simulink model "Adaptive_Control_KpKd"  (R2021b)
settings: Solver=VariableStepAuto  StartTime=0.0  StopTime=10  RelTol=1e-3
undefined symbols (not defined in the file or in its folder): coef_init, Kd, Kp, Kpi, Lambda, q_dq_init
(part 1 of 4)
settings Model: Creator=Yafei Ou  LastModifiedBy=ouyaf

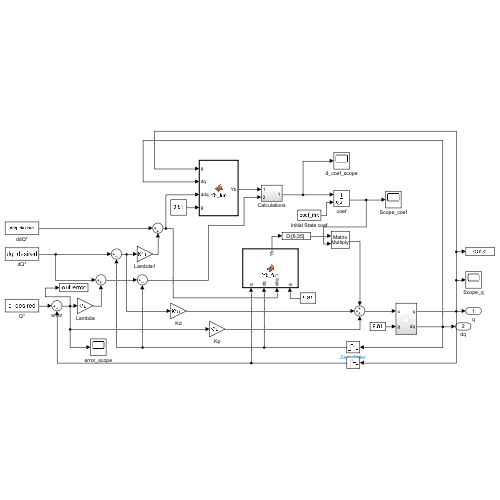
[thumbnail: Simulink's stored preview of the top-level diagram]
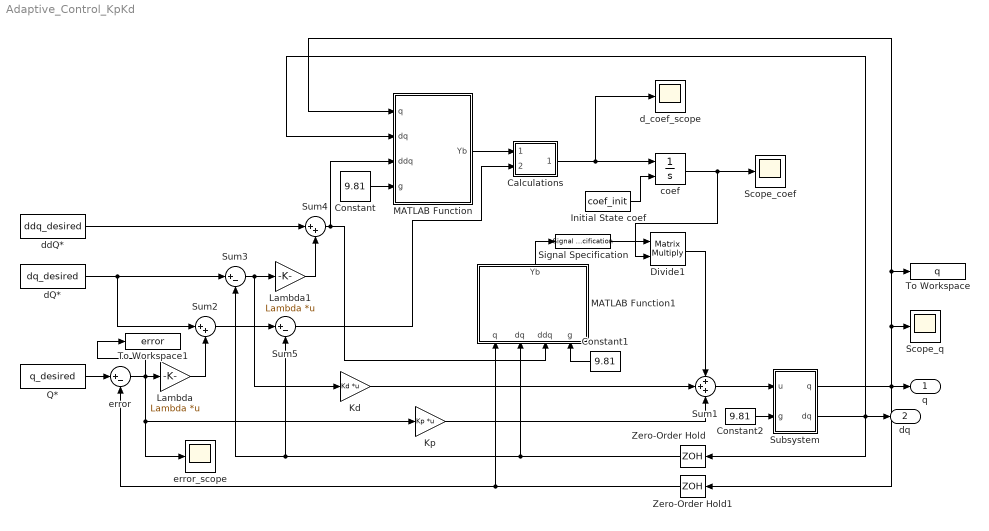
== system Adaptive_Control_KpKd ==
  Calculations : Subsystem
  Constant : Constant  Value=9.81
  Constant1 : Constant  Value=9.81
  Constant2 : Constant  Value=9.81
  Divide1 : Product  Multiplication=Matrix(*)
  Initial State coef : Constant  Value=coef_init
  Kd : Gain  Gain=Kd  Multiplication=Matrix(K*u)
  Kp : Gain  Gain=Kp  Multiplication=Matrix(K*u)
  Lambda : Gain  Gain=Lambda  Multiplication=Matrix(K*u)
  Lambda1 : Gain  Gain=Lambda  Multiplication=Matrix(K*u)
  MATLAB Function : MATLAB Function  TreatAsAtomicUnit=on
  MATLAB Function1 : MATLAB Function  TreatAsAtomicUnit=on
  Q* : FromWorkspace  VariableName=q_desired
  Scope_coef : Scope
  Scope_q : Scope
  Signal Specification : SignalSpecification  Dimensions=[6,35]
  Subsystem : Subsystem
  Sum1 : Sum  Inputs=+++
  Sum2 : Sum  Inputs=|++
  Sum3 : Sum  Inputs=|+-
  Sum4 : Sum  Inputs=|++
  Sum5 : Sum  Inputs=|+-
  To Workspace : ToWorkspace  VariableName=q  SaveFormat=Timeseries  SampleTime=-1
  To Workspace1 : ToWorkspace  VariableName=error  SaveFormat=Timeseries  SampleTime=-1
  Zero-Order Hold : ZeroOrderHold  SampleTime=0.001
  Zero-Order Hold1 : ZeroOrderHold  SampleTime=0.001
  coef : Integrator  InitialConditionSource=external
  dQ* : FromWorkspace  VariableName=dq_desired
  d_coef_scope : Scope
  ddQ* : FromWorkspace  VariableName=ddq_desired
  error : Sum  Inputs=|+-
  error_scope : Scope
  q : Outport
  dq : Outport  Port=2
  wires:
  Q*/1 -> error/1
  Constant/1 -> MATLAB Function/4(g)
  error/1 -> Kp/1, error_scope/1, Lambda/1, To Workspace1/1
  Lambda/1 -> Sum2/2
  dQ*/1 -> Sum2/1, Sum3/1
  Sum3/1 -> Kd/1, Lambda1/1
  ddQ*/1 -> Sum4/1
  Lambda1/1 -> Sum4/2
  Sum4/1 -> MATLAB Function/3(ddq), MATLAB Function1/3(ddq)
  Constant1/1 -> MATLAB Function1/4(g)
  Sum2/1 -> Sum5/1
  Kd/1 -> Sum1/2
  Signal Specification/1 -> Divide1/1
  Divide1/1 -> Sum1/1
  coef/1 -> Scope_coef/1, Divide1/2
  MATLAB Function1/1(Yb) -> Signal Specification/1
  Kp/1 -> Sum1/3
  Initial State coef/1 -> coef/2
  Zero-Order Hold/1 -> MATLAB Function1/2(dq), Sum5/2, Sum3/2
  Zero-Order Hold1/1 -> MATLAB Function1/1(q), error/2
  Subsystem/1(q) -> Scope_q/1, To Workspace/1, MATLAB Function/1(q), Zero-Order Hold1/1, q/1
  Subsystem/2(dq) -> MATLAB Function/2(dq), dq/1, Zero-Order Hold/1
  Sum1/1 -> Subsystem/1(u)
  Constant2/1 -> Subsystem/2(g)
  Calculations/1(Out1) -> d_coef_scope/1, coef/1
  MATLAB Function/1(Yb) -> Calculations/1(In1)
  Sum5/1 -> Calculations/2(In2)

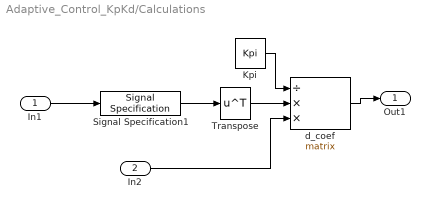
== system Adaptive_Control_KpKd/Calculations ==
  In1 : Inport
  In2 : Inport  Port=2
  Kpi : Constant  Value=Kpi
  Signal Specification1 : SignalSpecification  Dimensions=[6,35]
  Transpose : Math  Operator=transpose  SaturateOnIntegerOverflow=on
  d_coef : Product  Inputs=/**  Multiplication=Matrix(*)
  Out1 : Outport
  wires:
  Kpi/1 -> d_coef/1
  Transpose/1 -> d_coef/2
  In1/1 -> Signal Specification1/1
  Signal Specification1/1 -> Transpose/1
  d_coef/1 -> Out1/1
  In2/1 -> d_coef/3

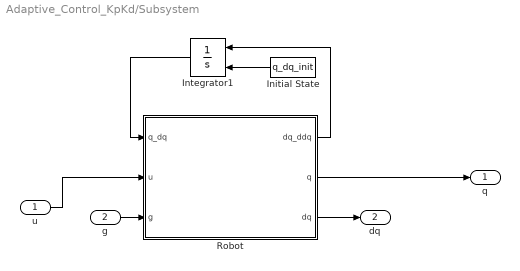
== system Adaptive_Control_KpKd/Subsystem ==
  u : Inport
  g : Inport  Port=2
  Initial State : Constant  Value=q_dq_init
  Integrator1 : Integrator  InitialConditionSource=external
  Robot : MATLAB Function  TreatAsAtomicUnit=on
  q : Outport
  dq : Outport  Port=2
  wires:
  Robot/1(dq_ddq) -> Integrator1/1
  Initial State/1 -> Integrator1/2
  u/1 -> Robot/2(u)
  Integrator1/1 -> Robot/1(q_dq)
  g/1 -> Robot/3(g)
  Robot/2(q) -> q/1
  Robot/3(dq) -> dq/1
